simulink model "gm_uz_6ph_spacevector_decode"  (R2024a)
settings: Solver=FixedStepDiscrete  StartTime=0.0  StopTime=350e-6  RelTol=1e-3
libraries: simulink x16, hdlsllib x3
settings Model: Creator=josef  LastModifiedBy=josef
settings SolverCC: AlgebraicLoopSolver=TrustRegion
settings DataIOCC: LimitDataPoints=on  SaveOutput=off  SaveTime=off
settings OptimizationCC: BlockReduction=off  ConditionallyExecuteInputs=off  DefaultParameterBehavior=Inlined  LifeSpan=inf
settings DebuggingCC: AlgebraicLoopMsg=error  InheritedTsInSrcMsg=none  SingleTaskRateTransMsg=error  UnconnectedInputMsg=warning  UnconnectedOutputMsg=warning  UnconnectedLineMsg=warning  AllowSymbolicDim=off  StrictBusMsg=ErrorOnBusTreatedAsVector  SFUnexpectedBacktrackingDiag=warning  SFNoUnconditionalDefaultTransitionDiag=warning  SFExecutionAtInitializationDiag=none  ArithmeticOperatorsInVariantConditions=warning
settings HardwareCC: ProdBitPerPointer=32  ProdBitPerSizeT=32  ProdBitPerPtrDiffT=32  ProdLargestAtomicFloat=None  ProdIntDivRoundTo=Undefined  ProdEndianess=Unspecified  ProdWordSize=32  ProdHWDeviceType=ASIC/FPGA->ASIC/FPGA  ProdEqTarget=off
settings ModelReferenceCC: EnableRefExpFcnMdlSchedulingChecks=on
settings SFSimCC: SimUseLocalCustomCode=off  CustomCodeUndefinedFunction=UseInterfaceOnly
settings RTWCC: RTWUseLocalCustomCode=off  GPUComputeCapability=3.5
settings CodeAppCC: StateflowObjectComments=on
settings GRTTargetCC: TargetLangStandard=C89/C90 (ANSI)
settings ConfigComp: CovScope=ReferencedModels  CovMetricSettings=dw  CovSaveCumulativeToWorkspaceVar=on  CovSaveSingleToWorkspaceVar=on  CovExternalEMLEnable=off  CovSFcnEnable=off

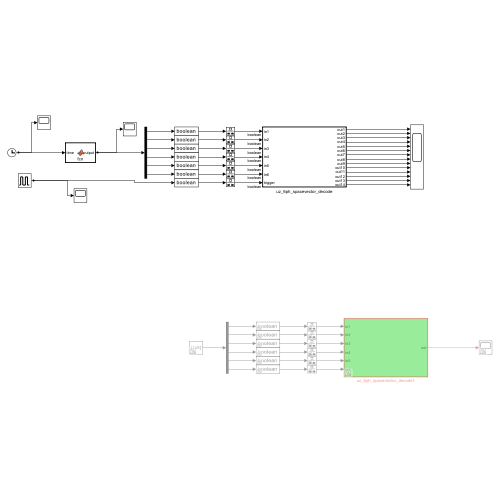
[thumbnail: Simulink's stored preview of the top-level diagram]
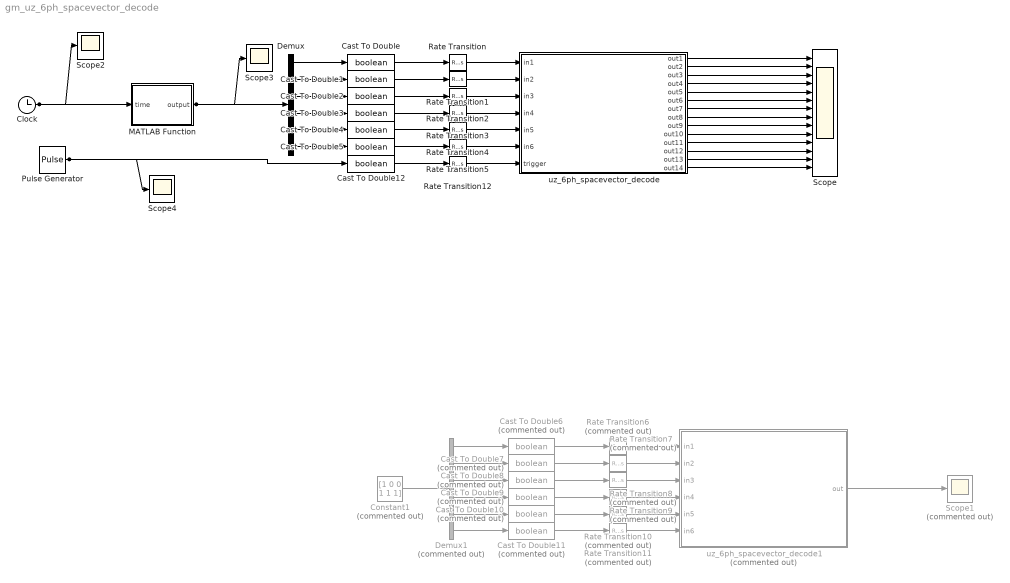
== system gm_uz_6ph_spacevector_decode ==
  Cast To Double{,1..5,12} (7 alike) : DataTypeConversion  OutDataTypeStr=boolean  SaturateOnIntegerOverflow=off  RndMeth=Floor
  Cast To Double{6..11} (6 alike) : DataTypeConversion  Commented=on  OutDataTypeStr=boolean  SaturateOnIntegerOverflow=off  RndMeth=Floor
  Clock : Clock
  Constant1 : Constant  Commented=on  Value=[1 0 0 1 1 1]
  Demux : Demux  Outputs=6
  Demux1 : Demux  Commented=on  Outputs=6
  MATLAB Function : MATLAB Function  TreatAsAtomicUnit=on
  Pulse Generator : DiscretePulseGenerator  PulseType=Time based  Period=100e-6  PulseWidth=5
  Rate Transition{,1..5,12} (7 alike) : RateTransition  OutPortSampleTime=1/100000000
  Rate Transition{6..11} (6 alike) : RateTransition  Commented=on  OutPortSampleTime=1/100000000
  Scope : Scope  NumInputPorts=14
  Scope1 : Scope  Commented=on
  Scope2 : Scope
  Scope3 : Scope
  Scope4 : Scope
  uz_6ph_spacevector_decode : Subsystem  TreatAsAtomicUnit=on
  uz_6ph_spacevector_decode1 : Subsystem  Commented=on  TreatAsAtomicUnit=on
  wires:
  Pulse Generator/1 -> Cast To Double12/1, Scope4/1
  Clock/1 -> MATLAB Function/1(time), Scope2/1
  Cast To Double12/1 -> Rate Transition12/1
  Rate Transition12/1 -> uz_6ph_spacevector_decode/7(trigger)
  uz_6ph_spacevector_decode/14(out14) -> Scope/14
  uz_6ph_spacevector_decode/13(out13) -> Scope/13
  uz_6ph_spacevector_decode/12(out12) -> Scope/12
  uz_6ph_spacevector_decode/11(out11) -> Scope/11
  uz_6ph_spacevector_decode/10(out10) -> Scope/10
  uz_6ph_spacevector_decode/9(out9) -> Scope/9
  uz_6ph_spacevector_decode/8(out8) -> Scope/8
  uz_6ph_spacevector_decode/7(out7) -> Scope/7
  uz_6ph_spacevector_decode/6(out6) -> Scope/6
  uz_6ph_spacevector_decode/5(out5) -> Scope/5
  uz_6ph_spacevector_decode/4(out4) -> Scope/4
  uz_6ph_spacevector_decode/3(out3) -> Scope/3
  uz_6ph_spacevector_decode/2(out2) -> Scope/2
  uz_6ph_spacevector_decode/1(out1) -> Scope/1
  Cast To Double7/1 -> Rate Transition7/1
  Cast To Double9/1 -> Rate Transition9/1
  Demux1/5 -> Cast To Double10/1
  Demux1/2 -> Cast To Double7/1
  Cast To Double6/1 -> Rate Transition6/1
  Demux1/4 -> Cast To Double9/1
  Demux1/3 -> Cast To Double8/1
  Cast To Double11/1 -> Rate Transition11/1
  Cast To Double8/1 -> Rate Transition8/1
  Rate Transition6/1 -> uz_6ph_spacevector_decode1/1(in1)
  Rate Transition8/1 -> uz_6ph_spacevector_decode1/3(in3)
  Rate Transition7/1 -> uz_6ph_spacevector_decode1/2(in2)
  Rate Transition9/1 -> uz_6ph_spacevector_decode1/4(in4)
  Cast To Double10/1 -> Rate Transition10/1
  Demux1/6 -> Cast To Double11/1
  uz_6ph_spacevector_decode1/1(out) -> Scope1/1
  Demux1/1 -> Cast To Double6/1
  Rate Transition10/1 -> uz_6ph_spacevector_decode1/5(in5)
  Constant1/1 -> Demux1/1
  Rate Transition11/1 -> uz_6ph_spacevector_decode1/6(in6)
  Rate Transition5/1 -> uz_6ph_spacevector_decode/6(in6)
  Rate Transition4/1 -> uz_6ph_spacevector_decode/5(in5)
  Rate Transition3/1 -> uz_6ph_spacevector_decode/4(in4)
  Rate Transition2/1 -> uz_6ph_spacevector_decode/3(in3)
  Rate Transition1/1 -> uz_6ph_spacevector_decode/2(in2)
  Rate Transition/1 -> uz_6ph_spacevector_decode/1(in1)
  MATLAB Function/1(output) -> Demux/1, Scope3/1
  Demux/6 -> Cast To Double5/1
  Demux/5 -> Cast To Double4/1
  Demux/4 -> Cast To Double3/1
  Demux/3 -> Cast To Double2/1
  Demux/2 -> Cast To Double1/1
  Demux/1 -> Cast To Double/1
  Cast To Double/1 -> Rate Transition/1
  Cast To Double1/1 -> Rate Transition1/1
  Cast To Double2/1 -> Rate Transition2/1
  Cast To Double3/1 -> Rate Transition3/1
  Cast To Double4/1 -> Rate Transition4/1
  Cast To Double5/1 -> Rate Transition5/1

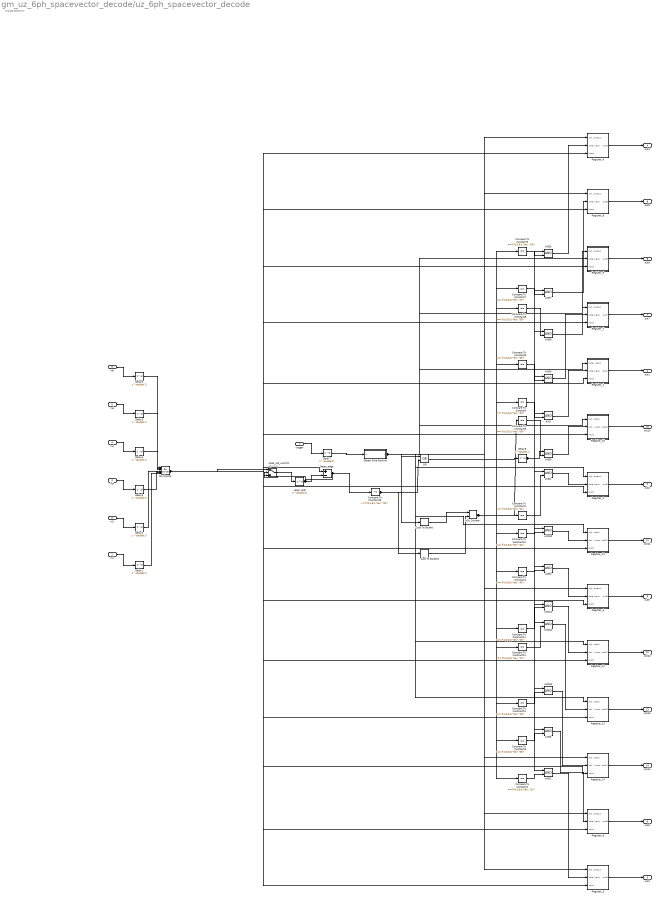
== system gm_uz_6ph_spacevector_decode/uz_6ph_spacevector_decode ==
  note: change detection
  in1 : Inport  OutDataTypeStr=boolean  PortDimensions=1  SampleTime=1e-08
  in2 : Inport  Port=2  OutDataTypeStr=boolean  PortDimensions=1  SampleTime=1e-08
  in3 : Inport  Port=3  OutDataTypeStr=boolean  PortDimensions=1  SampleTime=1e-08
  in4 : Inport  Port=4  OutDataTypeStr=boolean  PortDimensions=1  SampleTime=1e-08
  in5 : Inport  Port=5  OutDataTypeStr=boolean  PortDimensions=1  SampleTime=1e-08
  in6 : Inport  Port=6  OutDataTypeStr=boolean  PortDimensions=1  SampleTime=1e-08
  trigger : Inport  Port=7  OutDataTypeStr=boolean  PortDimensions=1  SampleTime=1e-08
  AND{,1..13} (14 alike) : Logic  AllPortsSameDT=off  OutDataTypeStr=boolean  SampleTime=1e-08
  Bit Concat : hdlsllib/Logic and Bit Operations/Bit Concat  numInputs=6
  Cast To Double : DataTypeConversion  OutDataTypeStr=boolean
  Cast To Double1 : DataTypeConversion  OutDataTypeStr=boolean
  Compare To Constant : simulink/Logic and Bit Operations/Compare To Constant  relop===  const="fi(0,0,8,0,\"hex\",\"00\")"  OutDataTypeStr=boolean
  Compare To Constant1 : simulink/Logic and Bit Operations/Compare To Constant  relop===  const="fi(0,0,8,0,\"hex\",\"01\")"  OutDataTypeStr=boolean
  Compare To Constant10 : simulink/Logic and Bit Operations/Compare To Constant  relop===  const="fi(0,0,8,0,\"hex\",\"0a\")"  OutDataTypeStr=boolean
  Compare To Constant11 : simulink/Logic and Bit Operations/Compare To Constant  relop===  const="fi(0,0,8,0,\"hex\",\"0b\")"  OutDataTypeStr=boolean
  Compare To Constant12 : simulink/Logic and Bit Operations/Compare To Constant  relop===  const="fi(0,0,8,0,\"hex\",\"0c\")"  OutDataTypeStr=boolean
  Compare To Constant13 : simulink/Logic and Bit Operations/Compare To Constant  relop===  const="fi(0,0,8,0,\"hex\",\"0d\")"  OutDataTypeStr=boolean
  Compare To Constant15 : simulink/Logic and Bit Operations/Compare To Constant  relop=~=  const="fi(0,1,8,0,\"hex\",\"00\")"  OutDataTypeStr=boolean
  Compare To Constant2 : simulink/Logic and Bit Operations/Compare To Constant  relop===  const="fi(0,0,8,0,\"hex\",\"02\")"  OutDataTypeStr=boolean
  Compare To Constant3 : simulink/Logic and Bit Operations/Compare To Constant  relop===  const="fi(0,0,8,0,\"hex\",\"03\")"  OutDataTypeStr=boolean
  Compare To Constant4 : simulink/Logic and Bit Operations/Compare To Constant  relop===  const="fi(0,0,8,0,\"hex\",\"04\")"  OutDataTypeStr=boolean
  Compare To Constant5 : simulink/Logic and Bit Operations/Compare To Constant  relop===  const="fi(0,0,8,0,\"hex\",\"05\")"  OutDataTypeStr=boolean
  Compare To Constant6 : simulink/Logic and Bit Operations/Compare To Constant  relop===  const="fi(0,0,8,0,\"hex\",\"06\")"  OutDataTypeStr=boolean
  Compare To Constant7 : simulink/Logic and Bit Operations/Compare To Constant  relop===  const="fi(0,0,8,0,\"hex\",\"07\")"  OutDataTypeStr=boolean
  Compare To Constant8 : simulink/Logic and Bit Operations/Compare To Constant  relop===  const="fi(0,0,8,0,\"hex\",\"08\")"  OutDataTypeStr=boolean
  Compare To Constant9 : simulink/Logic and Bit Operations/Compare To Constant  relop===  const="fi(0,0,8,0,\"hex\",\"09\")"  OutDataTypeStr=boolean
  Delay{1..8} (8 alike) : Delay  DelayLength=double(1)  InitialCondition=0  SampleTime=1e-08
  Detec_edge : Sum  Inputs=+-  OutDataTypeStr=int8  AccumDataTypeStr=int8  SampleTime=1e-08
  Detect Rise Positive : Subsystem  mask(Detect Rise Positive){vinit=double(0), InputProcessing=Elements as channels (sample based), OutDataTypeStr=boolean}
      mask prompts: vinit "Simulink:masks:InitialCondition_MP"; InputProcessing "Simulink:masks:InputProcessing_MP"; OutDataTypeStr "Simulink:masks:OutputDataType_MP"
      mask help: Simulink:masks:DetectRisePositive_MD
      mask init:
      | InputProcessing = 'Elements as channels (sample based)';
      | OutDataTypeStr = 'boolean';
      | vinit = double(0);
      mask TypeOptions InputProcessing: Simulink:masks:ColumnsAsChannelsFrameBased | Simulink:masks:ElementsAsChannelsSampleBased
      mask TypeOptions OutDataTypeStr: Simulink:masks:uint8 | Simulink:masks:boolean
      mask Display: fprintf('U > 0\n&  NOT\nU/z > 0')
  HDL Counter : hdlsllib/Sources/HDL Counter  CountType=Free running  CountInit=0  CountStep=1  CountMax=25  CountFromType=Initial value  CountFrom=0  CountResetPort=on  CountLoadPort=off  CountEnbPort=on  CountDirPort=off  CountHitOutputPort=off  CountDataType=Unsigned  CountWordLen=8  CountFracLen=0  CountSampTime=1
  OR : Logic  Operator=OR  AllPortsSameDT=off  OutDataTypeStr=boolean  SampleTime=1e-08
  Register_1 : Subsystem
  Register_10 : Subsystem
  Register_11 : Subsystem
  Register_12 : Subsystem
  Register_13 : Subsystem
  Register_14 : Subsystem
  Register_2 : Subsystem
  Register_3 : Subsystem
  Register_4 : Subsystem
  Register_5 : Subsystem
  Register_6 : Subsystem
  Register_7 : Subsystem
  Register_8 : Subsystem
  Register_9 : Subsystem
  reset_old2 : Delay  DelayLength=double(1)  InitialCondition=0  SampleTime=1e-08
  reset_old_switch1 : Switch  Criteria=u2 ~= 0  Threshold=double(0)  OutDataTypeStr=fixdt(0, 6, 0)  SampleTime=1e-08  SaturateOnIntegerOverflow=off  InputSameDT=off
  out1 : Outport  SampleTime=1e-08  VectorParamsAs1DForOutWhenUnconnected=off
  out2 : Outport  Port=2  SampleTime=1e-08  VectorParamsAs1DForOutWhenUnconnected=off
  out3 : Outport  Port=3  SampleTime=1e-08  VectorParamsAs1DForOutWhenUnconnected=off
  out4 : Outport  Port=4  SampleTime=1e-08  VectorParamsAs1DForOutWhenUnconnected=off
  out5 : Outport  Port=5  SampleTime=1e-08  VectorParamsAs1DForOutWhenUnconnected=off
  out6 : Outport  Port=6  SampleTime=1e-08  VectorParamsAs1DForOutWhenUnconnected=off
  out7 : Outport  Port=7  SampleTime=1e-08  VectorParamsAs1DForOutWhenUnconnected=off
  out8 : Outport  Port=8  SampleTime=1e-08  VectorParamsAs1DForOutWhenUnconnected=off
  out9 : Outport  Port=9  SampleTime=1e-08  VectorParamsAs1DForOutWhenUnconnected=off
  out10 : Outport  Port=10  SampleTime=1e-08  VectorParamsAs1DForOutWhenUnconnected=off
  out11 : Outport  Port=11  SampleTime=1e-08  VectorParamsAs1DForOutWhenUnconnected=off
  out12 : Outport  Port=12  SampleTime=1e-08  VectorParamsAs1DForOutWhenUnconnected=off
  out13 : Outport  Port=13  SampleTime=1e-08  VectorParamsAs1DForOutWhenUnconnected=off
  out14 : Outport  Port=14  SampleTime=1e-08  VectorParamsAs1DForOutWhenUnconnected=off
  wires:
  in1/1 -> Delay1/1
  in2/1 -> Delay2/1
  in3/1 -> Delay3/1
  in4/1 -> Delay4/1
  in5/1 -> Delay5/1
  in6/1 -> Delay6/1
  trigger/1 -> Delay7/1
  AND/1 -> Register_1/2(write input)
  AND1/1 -> Register_2/2(write input)
  AND10/1 -> Register_11/2(write input)
  AND11/1 -> Register_12/2(write input)
  AND12/1 -> Register_13/2(write input)
  AND13/1 -> Register_14/2(write input)
  AND2/1 -> Register_3/2(write input)
  AND3/1 -> Register_4/2(write input)
  AND4/1 -> Register_5/2(write input)
  AND5/1 -> Register_6/2(write input)
  AND6/1 -> Register_7/2(write input)
  AND7/1 -> Register_8/2(write input)
  AND8/1 -> Register_9/2(write input)
  AND9/1 -> Register_10/2(write input)
  Bit Concat/1 -> reset_old_switch1/1, Detec_edge/1, Register_14/3(input), Register_13/3(input), Register_12/3(input), Register_11/3(input), Register_10/3(input), Register_9/3(input), Register_8/3(input), Register_7/3(input), Register_6/3(input), Register_5/3(input), Register_4/3(input), Register_3/3(input), Register_2/3(input), Register_1/3(input)
  Cast To Double/1 -> HDL Counter/1
  Cast To Double1/1 -> HDL Counter/2
  Compare To Constant/1 -> AND/2
  Compare To Constant1/1 -> AND1/2
  Compare To Constant10/1 -> AND10/2
  Compare To Constant11/1 -> AND11/2
  Compare To Constant12/1 -> AND12/2
  Compare To Constant13/1 -> AND13/2
  Compare To Constant15/1 -> OR/2, Cast To Double1/1
  Compare To Constant2/1 -> AND2/2
  Compare To Constant3/1 -> AND3/2
  Compare To Constant4/1 -> AND4/2
  Compare To Constant5/1 -> AND5/2
  Compare To Constant6/1 -> AND6/2
  Compare To Constant7/1 -> AND7/2
  Compare To Constant8/1 -> AND8/2
  Compare To Constant9/1 -> AND9/2
  Delay1/1 -> Bit Concat/6
  Delay2/1 -> Bit Concat/5
  Delay3/1 -> Bit Concat/4
  Delay4/1 -> Bit Concat/3
  Delay5/1 -> Bit Concat/2
  Delay6/1 -> Bit Concat/1
  Delay7/1 -> Detect Rise Positive/1(U)
  Delay8/1 -> AND9/1, AND8/1, AND7/1, AND6/1, AND5/1, AND4/1, AND3/1, AND2/1, AND13/1, AND12/1, AND11/1, AND10/1, AND1/1, AND/1
  Detec_edge/1 -> reset_old_switch1/2, Compare To Constant15/1
  Detect Rise Positive/1(Y) -> OR/1, Cast To Double/1, Register_14/1(write output), Register_13/1(write output), Register_12/1(write output), Register_11/1(write output), Register_10/1(write output), Register_9/1(write output), Register_8/1(write output), Register_7/1(write output), Register_6/1(write output), Register_5/1(write output), Register_4/1(write output), Register_3/1(write output), Register_2/1(write output), Register_1/1(write output)
  HDL Counter/1 -> Compare To Constant9/1, Compare To Constant8/1, Compare To Constant7/1, Compare To Constant6/1, Compare To Constant5/1, Compare To Constant4/1, Compare To Constant3/1, Compare To Constant2/1, Compare To Constant13/1, Compare To Constant12/1, Compare To Constant11/1, Compare To Constant10/1, Compare To Constant1/1, Compare To Constant/1
  OR/1 -> Delay8/1
  Register_1/1(Out1) -> out1/1
  Register_10/1(out10) -> out10/1
  Register_11/1(out11) -> out11/1
  Register_12/1(out12) -> out12/1
  Register_13/1(out13) -> out13/1
  Register_14/1(out14) -> out14/1
  Register_2/1(out2) -> out2/1
  Register_3/1(out3) -> out3/1
  Register_4/1(out4) -> out4/1
  Register_5/1(out5) -> out5/1
  Register_6/1(out6) -> out6/1
  Register_7/1(out7) -> out7/1
  Register_8/1(out8) -> out8/1
  Register_9/1(out9) -> out9/1
  reset_old2/1 -> reset_old_switch1/3, Detec_edge/2
  reset_old_switch1/1 -> reset_old2/1

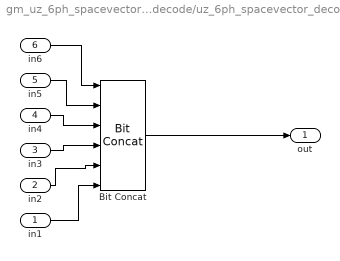
== system gm_uz_6ph_spacevector_decode/uz_6ph_spacevector_decode1 ==
  in1 : Inport
  in2 : Inport  Port=2
  in3 : Inport  Port=3
  in4 : Inport  Port=4
  in5 : Inport  Port=5
  in6 : Inport  Port=6
  Bit Concat : hdlsllib/Logic and Bit Operations/Bit Concat  numInputs=6
  out : Outport  VectorParamsAs1DForOutWhenUnconnected=off
  wires:
  Bit Concat/1 -> out/1
  in6/1 -> Bit Concat/1
  in5/1 -> Bit Concat/2
  in4/1 -> Bit Concat/3
  in3/1 -> Bit Concat/4
  in2/1 -> Bit Concat/5
  in1/1 -> Bit Concat/6

== system gm_uz_6ph_spacevector_decode/uz_6ph_spacevector_decode/Detect Rise Positive ==
  note: Edge
  note: U(k)
  U : Inport  OutDataTypeStr=boolean  SampleTime=1e-08
  Delay Input1 : UnitDelay  SampleTime=1e-08
  FixPt Relational Operator : RelationalOperator  Operator=>  OutDataTypeStr=boolean  SampleTime=1e-08  InputSameDT=off
  Positive : simulink/Logic and Bit Operations/Compare To Constant  relop=>  const=double(0)  OutDataTypeStr=boolean
  Y : Outport  SampleTime=1e-08
  wires:
  U/1 -> Positive/1
  Delay Input1/1 -> FixPt Relational Operator/2
  FixPt Relational Operator/1 -> Y/1
  Positive/1 -> FixPt Relational Operator/1, Delay Input1/1

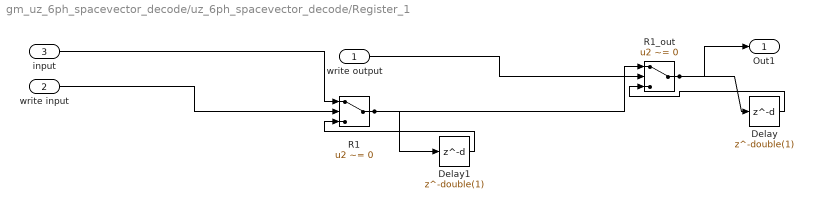
== system gm_uz_6ph_spacevector_decode/uz_6ph_spacevector_decode/Register_1 ==
  write output : Inport  OutDataTypeStr=boolean  PortDimensions=1  SampleTime=1e-08
  write input : Inport  Port=2  OutDataTypeStr=boolean  PortDimensions=1  SampleTime=1e-08
  input : Inport  Port=3  OutDataTypeStr=fixdt(0, 6, 0)  PortDimensions=1  SampleTime=1e-08
  Delay : Delay  DelayLength=double(1)  InitialCondition=0  SampleTime=1e-08
  Delay1 : Delay  DelayLength=double(1)  InitialCondition=0  SampleTime=1e-08
  R1 : Switch  Criteria=u2 ~= 0  Threshold=double(0)  OutDataTypeStr=int16  SampleTime=1e-08  SaturateOnIntegerOverflow=off  InputSameDT=off
  R1_out : Switch  Criteria=u2 ~= 0  Threshold=double(0)  OutDataTypeStr=fixdt(0, 6, 0)  SampleTime=1e-08  SaturateOnIntegerOverflow=off  InputSameDT=off
  Out1 : Outport  SampleTime=1e-08
  wires:
  write output/1 -> R1_out/2
  write input/1 -> R1/2
  input/1 -> R1/1
  Delay/1 -> R1_out/3
  Delay1/1 -> R1/3
  R1/1 -> R1_out/1, Delay1/1
  R1_out/1 -> Delay/1, Out1/1

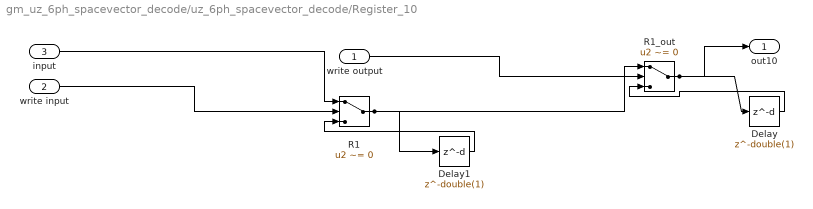
== system gm_uz_6ph_spacevector_decode/uz_6ph_spacevector_decode/Register_10 ==
  write output : Inport  OutDataTypeStr=boolean  PortDimensions=1  SampleTime=1e-08
  write input : Inport  Port=2  OutDataTypeStr=boolean  PortDimensions=1  SampleTime=1e-08
  input : Inport  Port=3  OutDataTypeStr=fixdt(0, 6, 0)  PortDimensions=1  SampleTime=1e-08
  Delay : Delay  DelayLength=double(1)  InitialCondition=0  SampleTime=1e-08
  Delay1 : Delay  DelayLength=double(1)  InitialCondition=0  SampleTime=1e-08
  R1 : Switch  Criteria=u2 ~= 0  Threshold=double(0)  OutDataTypeStr=int16  SampleTime=1e-08  SaturateOnIntegerOverflow=off  InputSameDT=off
  R1_out : Switch  Criteria=u2 ~= 0  Threshold=double(0)  OutDataTypeStr=fixdt(0, 6, 0)  SampleTime=1e-08  SaturateOnIntegerOverflow=off  InputSameDT=off
  out10 : Outport  SampleTime=1e-08
  wires:
  write output/1 -> R1_out/2
  write input/1 -> R1/2
  input/1 -> R1/1
  Delay/1 -> R1_out/3
  Delay1/1 -> R1/3
  R1/1 -> R1_out/1, Delay1/1
  R1_out/1 -> Delay/1, out10/1

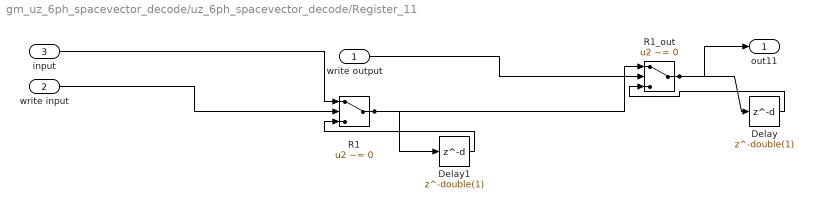
== system gm_uz_6ph_spacevector_decode/uz_6ph_spacevector_decode/Register_11 ==
  write output : Inport  OutDataTypeStr=boolean  PortDimensions=1  SampleTime=1e-08
  write input : Inport  Port=2  OutDataTypeStr=boolean  PortDimensions=1  SampleTime=1e-08
  input : Inport  Port=3  OutDataTypeStr=fixdt(0, 6, 0)  PortDimensions=1  SampleTime=1e-08
  Delay : Delay  DelayLength=double(1)  InitialCondition=0  SampleTime=1e-08
  Delay1 : Delay  DelayLength=double(1)  InitialCondition=0  SampleTime=1e-08
  R1 : Switch  Criteria=u2 ~= 0  Threshold=double(0)  OutDataTypeStr=int16  SampleTime=1e-08  SaturateOnIntegerOverflow=off  InputSameDT=off
  R1_out : Switch  Criteria=u2 ~= 0  Threshold=double(0)  OutDataTypeStr=fixdt(0, 6, 0)  SampleTime=1e-08  SaturateOnIntegerOverflow=off  InputSameDT=off
  out11 : Outport  SampleTime=1e-08
  wires:
  write output/1 -> R1_out/2
  write input/1 -> R1/2
  input/1 -> R1/1
  Delay/1 -> R1_out/3
  Delay1/1 -> R1/3
  R1/1 -> R1_out/1, Delay1/1
  R1_out/1 -> Delay/1, out11/1

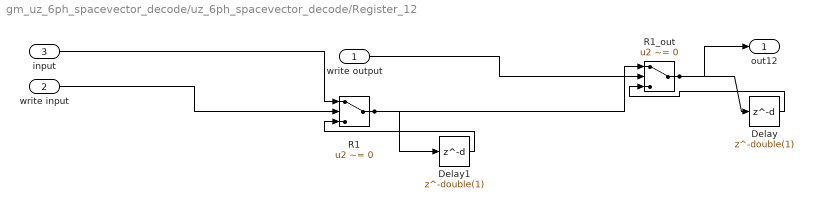
== system gm_uz_6ph_spacevector_decode/uz_6ph_spacevector_decode/Register_12 ==
  write output : Inport  OutDataTypeStr=boolean  PortDimensions=1  SampleTime=1e-08
  write input : Inport  Port=2  OutDataTypeStr=boolean  PortDimensions=1  SampleTime=1e-08
  input : Inport  Port=3  OutDataTypeStr=fixdt(0, 6, 0)  PortDimensions=1  SampleTime=1e-08
  Delay : Delay  DelayLength=double(1)  InitialCondition=0  SampleTime=1e-08
  Delay1 : Delay  DelayLength=double(1)  InitialCondition=0  SampleTime=1e-08
  R1 : Switch  Criteria=u2 ~= 0  Threshold=double(0)  OutDataTypeStr=int16  SampleTime=1e-08  SaturateOnIntegerOverflow=off  InputSameDT=off
  R1_out : Switch  Criteria=u2 ~= 0  Threshold=double(0)  OutDataTypeStr=fixdt(0, 6, 0)  SampleTime=1e-08  SaturateOnIntegerOverflow=off  InputSameDT=off
  out12 : Outport  SampleTime=1e-08
  wires:
  write output/1 -> R1_out/2
  write input/1 -> R1/2
  input/1 -> R1/1
  Delay/1 -> R1_out/3
  Delay1/1 -> R1/3
  R1/1 -> R1_out/1, Delay1/1
  R1_out/1 -> Delay/1, out12/1

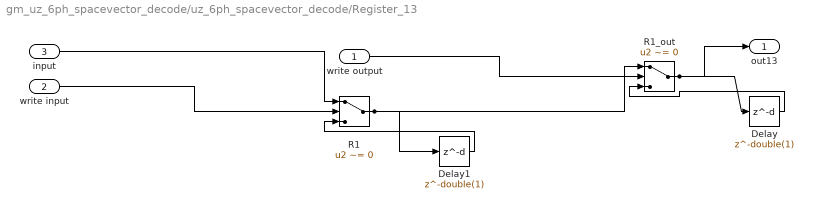
== system gm_uz_6ph_spacevector_decode/uz_6ph_spacevector_decode/Register_13 ==
  write output : Inport  OutDataTypeStr=boolean  PortDimensions=1  SampleTime=1e-08
  write input : Inport  Port=2  OutDataTypeStr=boolean  PortDimensions=1  SampleTime=1e-08
  input : Inport  Port=3  OutDataTypeStr=fixdt(0, 6, 0)  PortDimensions=1  SampleTime=1e-08
  Delay : Delay  DelayLength=double(1)  InitialCondition=0  SampleTime=1e-08
  Delay1 : Delay  DelayLength=double(1)  InitialCondition=0  SampleTime=1e-08
  R1 : Switch  Criteria=u2 ~= 0  Threshold=double(0)  OutDataTypeStr=int16  SampleTime=1e-08  SaturateOnIntegerOverflow=off  InputSameDT=off
  R1_out : Switch  Criteria=u2 ~= 0  Threshold=double(0)  OutDataTypeStr=fixdt(0, 6, 0)  SampleTime=1e-08  SaturateOnIntegerOverflow=off  InputSameDT=off
  out13 : Outport  SampleTime=1e-08
  wires:
  write output/1 -> R1_out/2
  write input/1 -> R1/2
  input/1 -> R1/1
  Delay/1 -> R1_out/3
  Delay1/1 -> R1/3
  R1/1 -> R1_out/1, Delay1/1
  R1_out/1 -> Delay/1, out13/1

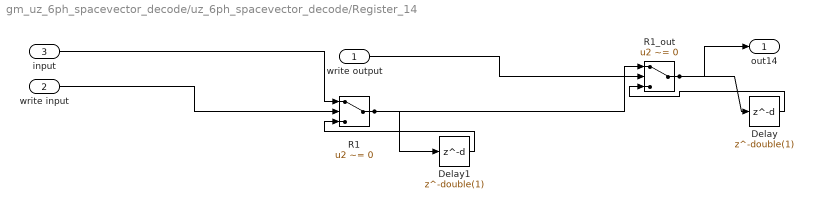
== system gm_uz_6ph_spacevector_decode/uz_6ph_spacevector_decode/Register_14 ==
  write output : Inport  OutDataTypeStr=boolean  PortDimensions=1  SampleTime=1e-08
  write input : Inport  Port=2  OutDataTypeStr=boolean  PortDimensions=1  SampleTime=1e-08
  input : Inport  Port=3  OutDataTypeStr=fixdt(0, 6, 0)  PortDimensions=1  SampleTime=1e-08
  Delay : Delay  DelayLength=double(1)  InitialCondition=0  SampleTime=1e-08
  Delay1 : Delay  DelayLength=double(1)  InitialCondition=0  SampleTime=1e-08
  R1 : Switch  Criteria=u2 ~= 0  Threshold=double(0)  OutDataTypeStr=int16  SampleTime=1e-08  SaturateOnIntegerOverflow=off  InputSameDT=off
  R1_out : Switch  Criteria=u2 ~= 0  Threshold=double(0)  OutDataTypeStr=fixdt(0, 6, 0)  SampleTime=1e-08  SaturateOnIntegerOverflow=off  InputSameDT=off
  out14 : Outport  SampleTime=1e-08
  wires:
  write output/1 -> R1_out/2
  write input/1 -> R1/2
  input/1 -> R1/1
  Delay/1 -> R1_out/3
  Delay1/1 -> R1/3
  R1/1 -> R1_out/1, Delay1/1
  R1_out/1 -> Delay/1, out14/1

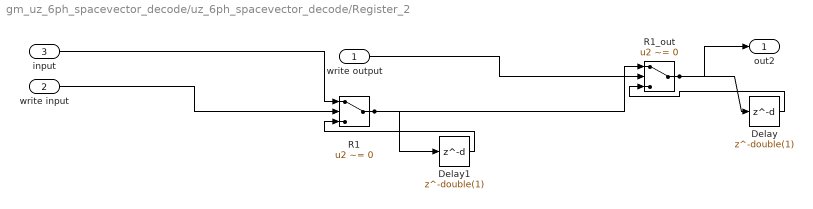
== system gm_uz_6ph_spacevector_decode/uz_6ph_spacevector_decode/Register_2 ==
  write output : Inport  OutDataTypeStr=boolean  PortDimensions=1  SampleTime=1e-08
  write input : Inport  Port=2  OutDataTypeStr=boolean  PortDimensions=1  SampleTime=1e-08
  input : Inport  Port=3  OutDataTypeStr=fixdt(0, 6, 0)  PortDimensions=1  SampleTime=1e-08
  Delay : Delay  DelayLength=double(1)  InitialCondition=0  SampleTime=1e-08
  Delay1 : Delay  DelayLength=double(1)  InitialCondition=0  SampleTime=1e-08
  R1 : Switch  Criteria=u2 ~= 0  Threshold=double(0)  OutDataTypeStr=int16  SampleTime=1e-08  SaturateOnIntegerOverflow=off  InputSameDT=off
  R1_out : Switch  Criteria=u2 ~= 0  Threshold=double(0)  OutDataTypeStr=fixdt(0, 6, 0)  SampleTime=1e-08  SaturateOnIntegerOverflow=off  InputSameDT=off
  out2 : Outport  SampleTime=1e-08
  wires:
  write output/1 -> R1_out/2
  write input/1 -> R1/2
  input/1 -> R1/1
  Delay/1 -> R1_out/3
  Delay1/1 -> R1/3
  R1/1 -> R1_out/1, Delay1/1
  R1_out/1 -> Delay/1, out2/1

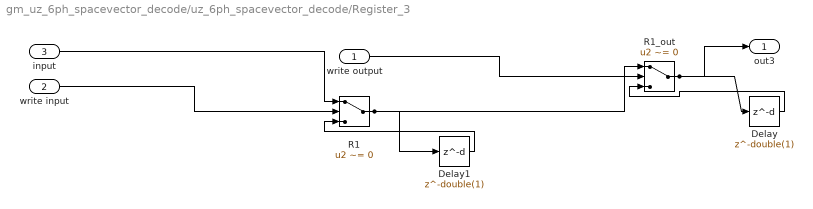
== system gm_uz_6ph_spacevector_decode/uz_6ph_spacevector_decode/Register_3 ==
  write output : Inport  OutDataTypeStr=boolean  PortDimensions=1  SampleTime=1e-08
  write input : Inport  Port=2  OutDataTypeStr=boolean  PortDimensions=1  SampleTime=1e-08
  input : Inport  Port=3  OutDataTypeStr=fixdt(0, 6, 0)  PortDimensions=1  SampleTime=1e-08
  Delay : Delay  DelayLength=double(1)  InitialCondition=0  SampleTime=1e-08
  Delay1 : Delay  DelayLength=double(1)  InitialCondition=0  SampleTime=1e-08
  R1 : Switch  Criteria=u2 ~= 0  Threshold=double(0)  OutDataTypeStr=int16  SampleTime=1e-08  SaturateOnIntegerOverflow=off  InputSameDT=off
  R1_out : Switch  Criteria=u2 ~= 0  Threshold=double(0)  OutDataTypeStr=fixdt(0, 6, 0)  SampleTime=1e-08  SaturateOnIntegerOverflow=off  InputSameDT=off
  out3 : Outport  SampleTime=1e-08
  wires:
  write output/1 -> R1_out/2
  write input/1 -> R1/2
  input/1 -> R1/1
  Delay/1 -> R1_out/3
  Delay1/1 -> R1/3
  R1/1 -> R1_out/1, Delay1/1
  R1_out/1 -> Delay/1, out3/1

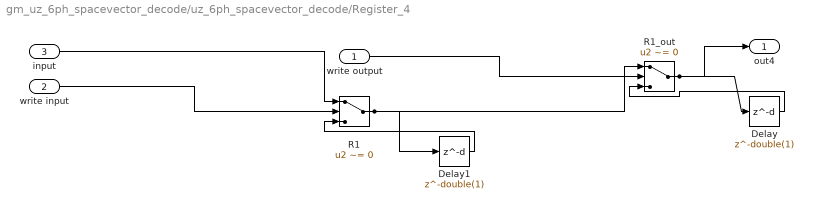
== system gm_uz_6ph_spacevector_decode/uz_6ph_spacevector_decode/Register_4 ==
  write output : Inport  OutDataTypeStr=boolean  PortDimensions=1  SampleTime=1e-08
  write input : Inport  Port=2  OutDataTypeStr=boolean  PortDimensions=1  SampleTime=1e-08
  input : Inport  Port=3  OutDataTypeStr=fixdt(0, 6, 0)  PortDimensions=1  SampleTime=1e-08
  Delay : Delay  DelayLength=double(1)  InitialCondition=0  SampleTime=1e-08
  Delay1 : Delay  DelayLength=double(1)  InitialCondition=0  SampleTime=1e-08
  R1 : Switch  Criteria=u2 ~= 0  Threshold=double(0)  OutDataTypeStr=int16  SampleTime=1e-08  SaturateOnIntegerOverflow=off  InputSameDT=off
  R1_out : Switch  Criteria=u2 ~= 0  Threshold=double(0)  OutDataTypeStr=fixdt(0, 6, 0)  SampleTime=1e-08  SaturateOnIntegerOverflow=off  InputSameDT=off
  out4 : Outport  SampleTime=1e-08
  wires:
  write output/1 -> R1_out/2
  write input/1 -> R1/2
  input/1 -> R1/1
  Delay/1 -> R1_out/3
  Delay1/1 -> R1/3
  R1/1 -> R1_out/1, Delay1/1
  R1_out/1 -> Delay/1, out4/1

== system gm_uz_6ph_spacevector_decode/uz_6ph_spacevector_decode/Register_5 ==
  write output : Inport  OutDataTypeStr=boolean  PortDimensions=1  SampleTime=1e-08
  write input : Inport  Port=2  OutDataTypeStr=boolean  PortDimensions=1  SampleTime=1e-08
  input : Inport  Port=3  OutDataTypeStr=fixdt(0, 6, 0)  PortDimensions=1  SampleTime=1e-08
  Delay : Delay  DelayLength=double(1)  InitialCondition=0  SampleTime=1e-08
  Delay1 : Delay  DelayLength=double(1)  InitialCondition=0  SampleTime=1e-08
  R1 : Switch  Criteria=u2 ~= 0  Threshold=double(0)  OutDataTypeStr=int16  SampleTime=1e-08  SaturateOnIntegerOverflow=off  InputSameDT=off
  R1_out : Switch  Criteria=u2 ~= 0  Threshold=double(0)  OutDataTypeStr=fixdt(0, 6, 0)  SampleTime=1e-08  SaturateOnIntegerOverflow=off  InputSameDT=off
  out5 : Outport  SampleTime=1e-08
  wires:
  write output/1 -> R1_out/2
  write input/1 -> R1/2
  input/1 -> R1/1
  Delay/1 -> R1_out/3
  Delay1/1 -> R1/3
  R1/1 -> R1_out/1, Delay1/1
  R1_out/1 -> Delay/1, out5/1

== system gm_uz_6ph_spacevector_decode/uz_6ph_spacevector_decode/Register_6 ==
  write output : Inport  OutDataTypeStr=boolean  PortDimensions=1  SampleTime=1e-08
  write input : Inport  Port=2  OutDataTypeStr=boolean  PortDimensions=1  SampleTime=1e-08
  input : Inport  Port=3  OutDataTypeStr=fixdt(0, 6, 0)  PortDimensions=1  SampleTime=1e-08
  Delay : Delay  DelayLength=double(1)  InitialCondition=0  SampleTime=1e-08
  Delay1 : Delay  DelayLength=double(1)  InitialCondition=0  SampleTime=1e-08
  R1 : Switch  Criteria=u2 ~= 0  Threshold=double(0)  OutDataTypeStr=int16  SampleTime=1e-08  SaturateOnIntegerOverflow=off  InputSameDT=off
  R1_out : Switch  Criteria=u2 ~= 0  Threshold=double(0)  OutDataTypeStr=fixdt(0, 6, 0)  SampleTime=1e-08  SaturateOnIntegerOverflow=off  InputSameDT=off
  out6 : Outport  SampleTime=1e-08
  wires:
  write output/1 -> R1_out/2
  write input/1 -> R1/2
  input/1 -> R1/1
  Delay/1 -> R1_out/3
  Delay1/1 -> R1/3
  R1/1 -> R1_out/1, Delay1/1
  R1_out/1 -> Delay/1, out6/1

== system gm_uz_6ph_spacevector_decode/uz_6ph_spacevector_decode/Register_7 ==
  write output : Inport  OutDataTypeStr=boolean  PortDimensions=1  SampleTime=1e-08
  write input : Inport  Port=2  OutDataTypeStr=boolean  PortDimensions=1  SampleTime=1e-08
  input : Inport  Port=3  OutDataTypeStr=fixdt(0, 6, 0)  PortDimensions=1  SampleTime=1e-08
  Delay : Delay  DelayLength=double(1)  InitialCondition=0  SampleTime=1e-08
  Delay1 : Delay  DelayLength=double(1)  InitialCondition=0  SampleTime=1e-08
  R1 : Switch  Criteria=u2 ~= 0  Threshold=double(0)  OutDataTypeStr=int16  SampleTime=1e-08  SaturateOnIntegerOverflow=off  InputSameDT=off
  R1_out : Switch  Criteria=u2 ~= 0  Threshold=double(0)  OutDataTypeStr=fixdt(0, 6, 0)  SampleTime=1e-08  SaturateOnIntegerOverflow=off  InputSameDT=off
  out7 : Outport  SampleTime=1e-08
  wires:
  write output/1 -> R1_out/2
  write input/1 -> R1/2
  input/1 -> R1/1
  Delay/1 -> R1_out/3
  Delay1/1 -> R1/3
  R1/1 -> R1_out/1, Delay1/1
  R1_out/1 -> Delay/1, out7/1

== system gm_uz_6ph_spacevector_decode/uz_6ph_spacevector_decode/Register_8 ==
  write output : Inport  OutDataTypeStr=boolean  PortDimensions=1  SampleTime=1e-08
  write input : Inport  Port=2  OutDataTypeStr=boolean  PortDimensions=1  SampleTime=1e-08
  input : Inport  Port=3  OutDataTypeStr=fixdt(0, 6, 0)  PortDimensions=1  SampleTime=1e-08
  Delay : Delay  DelayLength=double(1)  InitialCondition=0  SampleTime=1e-08
  Delay1 : Delay  DelayLength=double(1)  InitialCondition=0  SampleTime=1e-08
  R1 : Switch  Criteria=u2 ~= 0  Threshold=double(0)  OutDataTypeStr=int16  SampleTime=1e-08  SaturateOnIntegerOverflow=off  InputSameDT=off
  R1_out : Switch  Criteria=u2 ~= 0  Threshold=double(0)  OutDataTypeStr=fixdt(0, 6, 0)  SampleTime=1e-08  SaturateOnIntegerOverflow=off  InputSameDT=off
  out8 : Outport  SampleTime=1e-08
  wires:
  write output/1 -> R1_out/2
  write input/1 -> R1/2
  input/1 -> R1/1
  Delay/1 -> R1_out/3
  Delay1/1 -> R1/3
  R1/1 -> R1_out/1, Delay1/1
  R1_out/1 -> Delay/1, out8/1

== system gm_uz_6ph_spacevector_decode/uz_6ph_spacevector_decode/Register_9 ==
  write output : Inport  OutDataTypeStr=boolean  PortDimensions=1  SampleTime=1e-08
  write input : Inport  Port=2  OutDataTypeStr=boolean  PortDimensions=1  SampleTime=1e-08
  input : Inport  Port=3  OutDataTypeStr=fixdt(0, 6, 0)  PortDimensions=1  SampleTime=1e-08
  Delay : Delay  DelayLength=double(1)  InitialCondition=0  SampleTime=1e-08
  Delay1 : Delay  DelayLength=double(1)  InitialCondition=0  SampleTime=1e-08
  R1 : Switch  Criteria=u2 ~= 0  Threshold=double(0)  OutDataTypeStr=int16  SampleTime=1e-08  SaturateOnIntegerOverflow=off  InputSameDT=off
  R1_out : Switch  Criteria=u2 ~= 0  Threshold=double(0)  OutDataTypeStr=fixdt(0, 6, 0)  SampleTime=1e-08  SaturateOnIntegerOverflow=off  InputSameDT=off
  out9 : Outport  SampleTime=1e-08
  wires:
  write output/1 -> R1_out/2
  write input/1 -> R1/2
  input/1 -> R1/1
  Delay/1 -> R1_out/3
  Delay1/1 -> R1/3
  R1/1 -> R1_out/1, Delay1/1
  R1_out/1 -> Delay/1, out9/1

== matlab function gm_uz_6ph_spacevector_decode/MATLAB Function ==
  data: time input; output output
function output = fcn(time)

% output_ar = [
% 1,0,0,0,0,0;    
% 0,1,0,0,0,0;
% 1,1,0,0,0,0;
% 0,0,1,0,0,0;
% 1,0,1,0,0,0;
% 0,1,1,0,0,0;
% 1,1,1,0,0,0;
% 0,0,0,1,0,0;
% 1,0,0,1,0,0;
% 0,1,0,1,0,0;
% 1,1,0,1,0,0;
% 0,0,1,1,0,0;
% 1,0,1,1,0,0;
% 0,1,1,1,0,0;
% 
% 1,1,1,0,0,0; 
% 1,0,0,0,0,0;    
% 0,1,0,0,0,0;
% 1,1,0,0,0,0;
% 0,0,1,0,0,0;
% 1,0,1,0,0,0;
% 0,1,1,0,0,0;
% 1,1,1,0,0,0;
% 0,0,0,1,0,0;
% 1,0,0,1,0,0;
% 0,1,0,1,0,0;
% 1,1,0,1,0,0;
% 0,0,1,1,0,0;
% 1,0,1,1,0,0;
% 
% 0,1,1,1,0,0;
% 1,1,1,1,1,0; 
% 1,0,0,0,0,0;    
% 0,1,0,0,0,0;
% 1,1,0,0,0,0;
% 0,0,1,0,0,0;
% 1,0,1,0,0,0;
% 0,1,1,0,0,0;
% 1,1,1,0,0,0;
% 0,0,0,1,0,0;
% 1,0,0,1,0,0;
% 0,1,0,1,0,0;
% 1,1,0,1,0,0;
% 0,0,1,1,0,0;
% 
% 1,0,1,1,0,0;
% 0,1,1,1,0,0;
% ];
% 
% time_output_ar = [[1:1:14]*2e-6, [1:1:14]*2e-6+105e-6, [1:1:14]*2e-6+205e-6];


output_ar = [
0,0,0,0,0,0;
1,0,0,0,0,0;    
0,1,0,0,0,0;
1,1,0,0,0,0;
0,1,0,0,0,0;
1,0,0,0,0,0;  
0,0,0,0,0,0;

0,0,0,0,0,1;
1,0,0,0,0,1;    
0,1,0,0,0,1;
1,1,0,0,0,1;
0,1,0,0,0,1;
1,0,0,0,0,1;
0,0,0,0,0,1;

0,0,0,0,0,0;
1,0,0,0,0,0;    
0,1,0,0,0,0;
1,1,0,0,0,0;
0,1,0,0,0,0;
1,0,0,0,0,0;
0,0,0,0,0,0;
];

time_output_ar = [[1:1:7]*10e-6, [1:1:7]*10e-6+100e-6, [1:1:7]*10e-6+200e-6 ];



idx = 1;
for i = 1:1:length(time_output_ar)
    if time > time_output_ar(i)
        idx = i;
    end
end

output = output_ar(idx,:);
